simulink model "Pendulo_Invertido"  (R2025b)
settings: Solver=ode45  StartTime=0.0  StopTime=10.0  MaxStep=1e-3  RelTol=1e-3
values from neighbouring files (symbols this model uses):
  alpha = m_p + m_c    (= 2.1)    [Coefficients.m]
  b = 2*zeta_c*omega_p*alpha    [Coefficients.m]
  beta = 2*zeta_p*omega_p*(lambda-mu^2/alpha)    [Coefficients.m]
  F_equilibrium = 1.5*alpha*g*tand(80)    [Coefficients.m]
  g = 9.80665    [Coefficients.m]
  h_c = 0.05    [Coefficients.m]
  l = 0.5    [Coefficients.m]
  lambda = 4/3 * m_p * l^2    (= 0.0333333333333)    [Coefficients.m]
  mu = m_p * l    (= 0.05)    [Coefficients.m]
  x_ref = 0    [Coefficients.m]
libraries: sim3dlib x4, fuzblock x2
settings Model: SimulationMode=accelerator  Creator=barrios14101  LastModifiedBy=admin

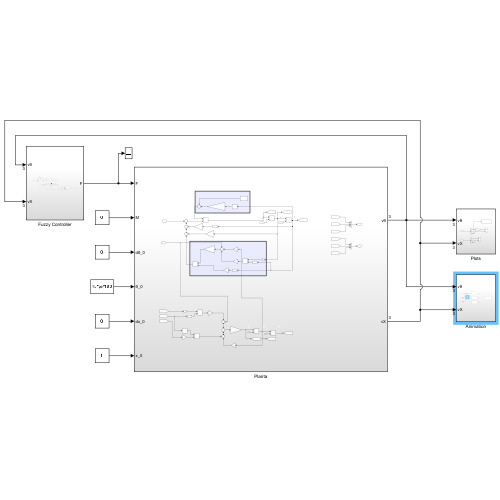
[thumbnail: Simulink's stored preview of the top-level diagram]
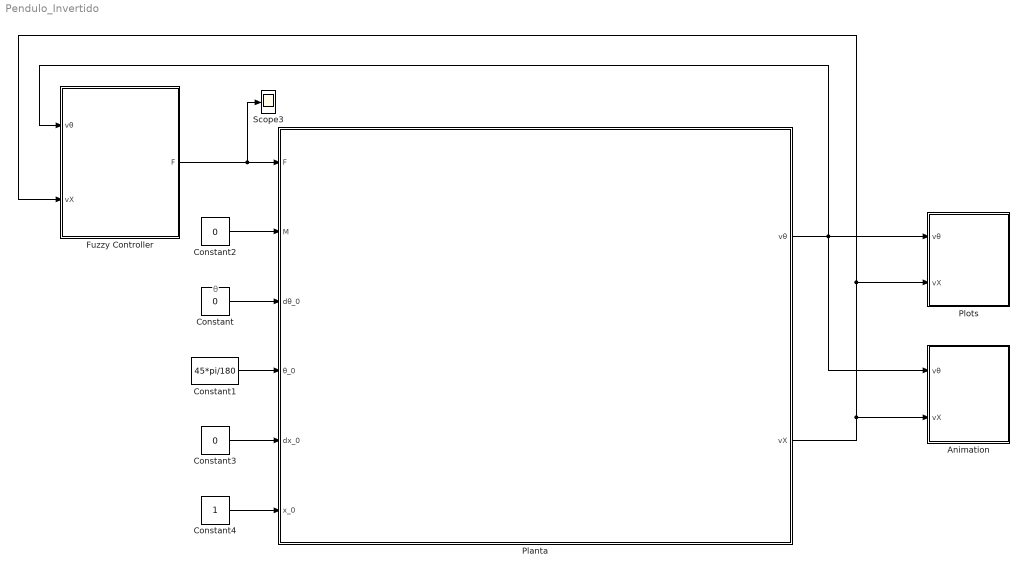
== system Pendulo_Invertido ==
  note: θ
  Animation : Subsystem
  Constant : Constant  Value=0
  Constant1 : Constant  Value=45*pi/180
  Constant2 : Constant  Value=0
  Constant3 : Constant  Value=0
  Constant4 : Constant
  Fuzzy Controller : Subsystem
  Planta : Subsystem
  Plots : Subsystem
  Scope3 : Scope
      settings: ActiveDisplayYMinimum=-600.8821467974509  ActiveDisplayYMaximum=220.63357171688955  DataLoggingDecimation=50  DataLoggingVariableName=ScopeData2
  wires:
  Planta/1(vθ) -> Animation/1(vθ), Plots/1(vθ), Fuzzy Controller/1(vθ)
  Constant/1 -> Planta/3(dθ_0)
  Constant1/1 -> Planta/4(θ_0)
  Planta/2(vX) -> Fuzzy Controller/2(vX), Plots/2(vX), Animation/2(vX)
  Fuzzy Controller/1(F) -> Scope3/1, Planta/1(F)
  Constant2/1 -> Planta/2(M)
  Constant3/1 -> Planta/5(dx_0)
  Constant4/1 -> Planta/6(x_0)

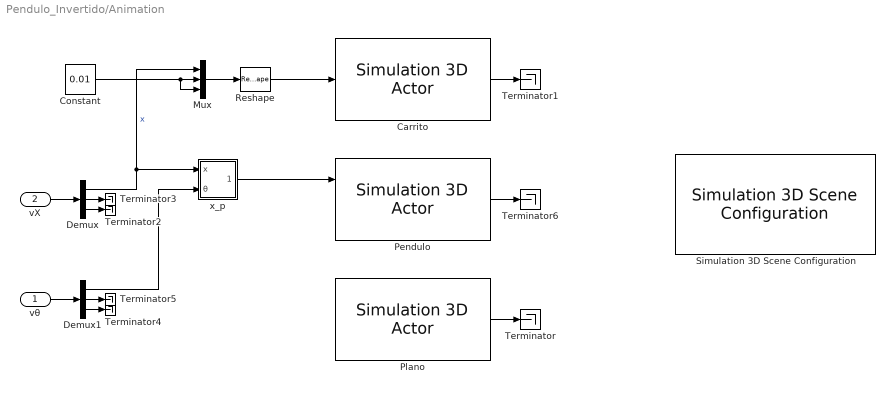
== system Pendulo_Invertido/Animation ==
  vθ : Inport
  vX : Inport  Port=2
  Carrito : sim3dlib/Simulation 3D Actor  Priority=1  ActorName=Carrito  ParentName=Scene Origin  Operation=Create at setup  InitScriptText=|  SampleTime=-1  Translation=[0 0 0]  Rotation=[0 0 0]  Scale=[1 1 1]  InputsText=Carrito.Translation  aMode=5  ActorTag=Carrito  ActorType=Sim3dActor  ID=C
      | createShape(Actor, 'box', [0.5 0.2 0.2]);
      | Actor.Color = [1 0 0];
      | Actor.Physics = false;
      | Actor.Gravity = false;
      | 
      | % Reserved keywords:
      | % - Actor : handle to this actor object
      | % - World : handle to the world object
      | 
      | % Examples:
      | 
      | % Create a primitive geometry (optional)
      | % createShape(Actor, 'box', [1 1 1]);
      | 
      | % Initialize values (optional)
      | % Actor.Physics = true;
      | % Actor.Color = [1 0 0];
  Constant : Constant  Value=0.01
  Demux : Demux  Outputs=3
  Demux1 : Demux  Outputs=3
  Mux : Mux  Inputs=3
  Pendulo : sim3dlib/Simulation 3D Actor  Priority=1  ActorName=Pendulo  ParentName=Scene Origin  Operation=Create at setup  InitScriptText=|  SampleTime=-1  Translation=[0 0 0]  Rotation=[0 0 0]  Scale=[1 1 1]  InputsText=Pendulo.Translation Pendulo.Rotation  aMode=5  ActorTag=Pendulo  ActorType=Sim3dActor  ID=C
      | createShape(Actor, 'cylinder', [0.025 0.025 0.1]);Actor.Color = [1 0 0];
      | Actor.Physics = false;
      | Actor.Gravity = false;
      | 
      | % Reserved keywords:
      | % - Actor : handle to this actor object
      | % - World : handle to the world object
      | 
      | % Examples:
      | 
      | % Create a primitive geometry (optional)
      | % createShape(Actor, 'box', [1 1 1]);
      | 
      | % Initialize values (optional)
      | % Actor.Physics = true;
      | % Actor.Color = [1 0 0];
  Plano : sim3dlib/Simulation 3D Actor  Priority=1  ActorName=Sim3dActor1  ParentName=Scene Origin  Operation=Create at setup  InitScriptText=|  SampleTime=-1  Translation=[0 0 0]  Rotation=[0 0 0]  Scale=[1 1 1]  aMode=5  ActorTag=Sim3dActor1  ActorType=Sim3dActor  ID=1
      | createShape(Actor, 'plane', [5 5 0.1]);
      | Actor.PreciseContacts = true;
  Reshape : Reshape  OutputDimensionality=Column vector (2-D)
  Simulation 3D Scene Configuration : sim3dlib/Simulation 3D Scene Configuration  Priority=0  ProjectFormat=Default Scenes  SceneDesc=Empty scene  ProjectName=C:\Program Files\MATLAB\R2025b\toolbox\shared\sim3d_projects\automotive_project_windows\UE\WindowsNoEditor\VehicleSimulation.exe  ScenePath=/Game/Maps/HwStrght  EnableOpenDRIVE=off  vehTagList={'Carrito';'Custom';'Scene Origin';'Sim3dActor1'}  vehTag=Carrito  AttachedCameraRelativeTranslation=[0 0 0]  FreeCameraDefaultInitialTranslation=[-6, 0, 2]  AttachedCameraRelativeRotation=[0 0 0]  FreeCameraDefaultInitialRotation=[0, -15, 0]  ViewpointName=Custom  FreeCameraInitialTranslation=[0, 0, 0]  ViewpointTranslation=[0 0 0]  FreeCameraInitialRotation=[0, 0, 0]  ViewpointRotation=[0 0 0]  OpVisEn=off  Ts=.02  EnableWindow=on  EnableRemoteAccess=off  EnableWeather=off  SunAzimuth=90  SunAltitude=40.0  EnableGeospatialSun=off  Latitude=0  Longitude=0  Date=2023-01-01  Time=10:30:00  GeoTimeZone=-5.0  SunDaylightSaving=off  wind=1  clouds=10  EnableVolumetricClouds=off  CloudCoverage=0  CloudAltitude=6  fog=0  rain=0  RaindropsEffect=off  SnowDensity=0  EnableGeospatial=off  TilesetSource=Earth terrain  UseTrueOrigin=off  OriginHeight=200  OriginLatitude=40.744652  OriginLongitude=-73.988864  MapStyle=Aerial  AdditionalAssetIDs=[]  UseAdvancedSunSky=off  SolarTime=11  TimeZone=-5  Day=21  Month=9  Year=2022  UseDaylightSavingTime=on  DSTStartDay=10  DSTStartMonth=3  DSTEndDay=3  DSTEndMonth=11  DSTSwitchHour=2  sensorTag=MainCamera1  sensorId=1  sensorName=MainCamera1  mountLoc=Origin  offsetFlag=off  tmountOffset=[0, 0, 0]  rmountOffset=[0, 0, 0]  HorizontalResolution=1280  VerticalResolution=720  HorizontalFOV=60  mountPoint=[0 0 0]  mountOrientation=[0 0 0]  aMode=5  ID=1  GeoTrigger=Inactive  ViewNameList={'Custom'}  ViewTranslationList={'[0 0 0]'}  ViewRotationList={'[0 0 0]'}
      settings: LibrarySourceBlock=sl3dlib/Simulation 3D/Environment/Simulation 3D Scene Configuration
  Terminator{,1..6} (7 alike) : Terminator
  x_p : Subsystem  TreatAsAtomicUnit=on
  wires:
  Plano/1 -> Terminator/1
  Carrito/1 -> Terminator1/1
  vX/1 -> Demux/1
  Demux/3 -> Terminator2/1
  Demux/2 -> Terminator3/1
  Demux1/3 -> Terminator4/1
  Demux1/2 -> Terminator5/1
  vθ/1 -> Demux1/1
  Constant/1 -> Mux/3, Mux/2
  Demux/1 -> Mux/1, x_p/1(x)  "x"
  Mux/1 -> Reshape/1
  Pendulo/1 -> Terminator6/1
  Demux1/1 -> x_p/2(θ)
  x_p/1(vX_p) -> Pendulo/1
  Reshape/1 -> Carrito/1

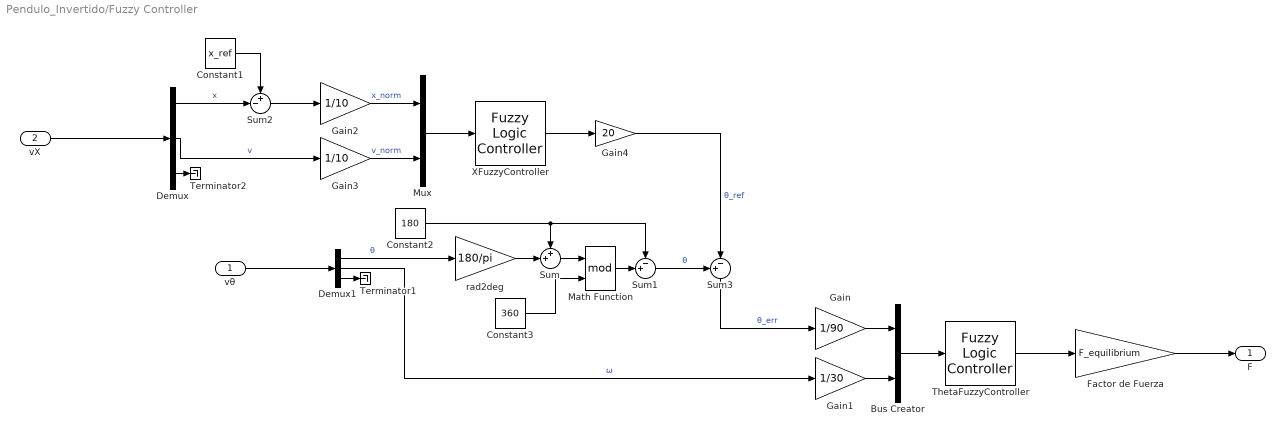
== system Pendulo_Invertido/Fuzzy Controller ==
  vθ : Inport
  vX : Inport  Port=2
  Bus Creator : BusCreator  Inputs=2
  Constant1 : Constant  Value=x_ref
  Constant2 : Constant  Value=180
  Constant3 : Constant  Value=360
  Demux : Demux  Outputs=3
  Demux1 : Demux  Outputs=3
  Factor de Fuerza : Gain  Gain=F_equilibrium
  Gain : Gain  Gain=1/90
  Gain1 : Gain  Gain=1/30
  Gain2 : Gain  Gain=1/10
  Gain3 : Gain  Gain=1/10
  Gain4 : Gain  Gain=20
  Math Function : Math  Operator=mod  OutputSignalType=real
  Mux : Mux  Inputs=2
  Sum : Sum  Inputs=++|
  Sum1 : Sum  Inputs=-+|
  Sum2 : Sum  Inputs=+-|
  Sum3 : Sum  Inputs=+-|
  Terminator1 : Terminator
  Terminator2 : Terminator
  ThetaFuzzyController : fuzblock/Fuzzy Logic  Controller  FIS='ThetaFuzzyController.fis'  OutputSampleNumber=101  DataType=double  UseLookupTable=off  NumBreakpoints=10  FuzzifiedInputs=off  RuleFiringStrengths=off  RuleOutputs=off  AggregatedOutputs=off  SimulateUsing=Interpreted execution  OutOfRangeInputValueMessage=warning  NoRuleFiredMessage=warning  EmptyOutputFuzzySetMessage=warning
  XFuzzyController : fuzblock/Fuzzy Logic  Controller  FIS='XFuzzyController.fis'  OutputSampleNumber=101  DataType=double  UseLookupTable=off  NumBreakpoints=10  FuzzifiedInputs=off  RuleFiringStrengths=off  RuleOutputs=off  AggregatedOutputs=off  SimulateUsing=Interpreted execution  OutOfRangeInputValueMessage=warning  NoRuleFiredMessage=warning  EmptyOutputFuzzySetMessage=warning
  rad2deg : Gain  Gain=180/pi
  F : Outport
  wires:
  ThetaFuzzyController/1 -> Factor de Fuerza/1
  Constant2/1 -> Sum1/1, Sum/1
  rad2deg/1 -> Sum/2
  Math Function/1 -> Sum1/2
  Demux1/2 -> Gain1/1  "ω"
  vθ/1 -> Demux1/1
  Bus Creator/1 -> ThetaFuzzyController/1
  Demux1/1 -> rad2deg/1  "θ"
  Sum/1 -> Math Function/1
  Gain1/1 -> Bus Creator/2
  Constant3/1 -> Math Function/2
  Gain/1 -> Bus Creator/1
  vX/1 -> Demux/1
  Gain2/1 -> Mux/1  "x_norm"
  Demux/2 -> Gain3/1  "v"
  Gain3/1 -> Mux/2  "v_norm"
  Mux/1 -> XFuzzyController/1
  XFuzzyController/1 -> Gain4/1
  Sum1/1 -> Sum3/1  "θ"
  Demux/1 -> Sum2/2  "x"
  Constant1/1 -> Sum2/1
  Sum2/1 -> Gain2/1
  Gain4/1 -> Sum3/2  "θ_ref"
  Sum3/1 -> Gain/1  "θ_err"
  Factor de Fuerza/1 -> F/1
  Demux1/3 -> Terminator1/1
  Demux/3 -> Terminator2/1

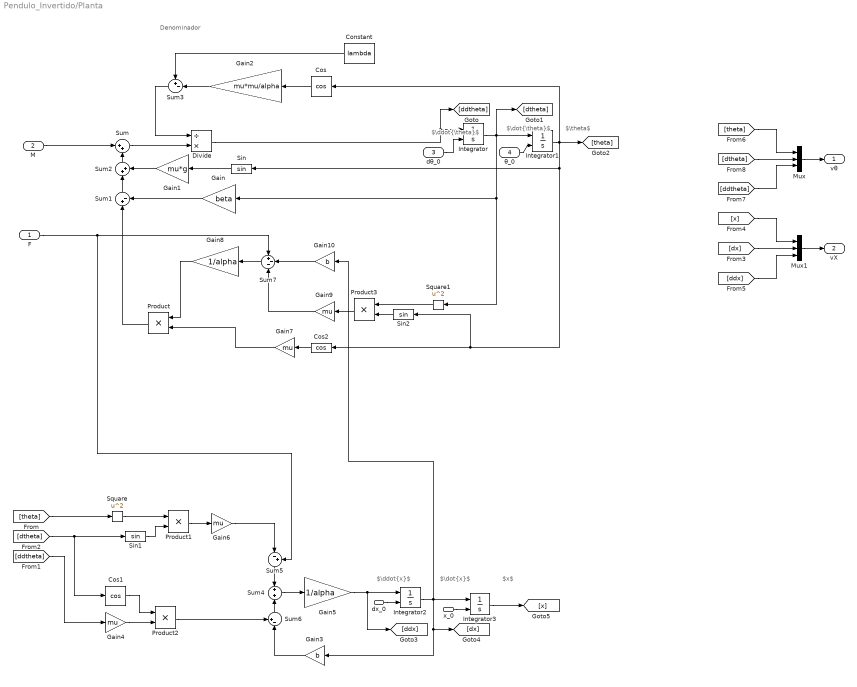
== system Pendulo_Invertido/Planta ==
  note: Denominador
  note: $\ddot{\theta}$
  note: $\dot{\theta}$
  note: $\theta$
  note: $x$
  note: $\ddot{x}$
  note: $\dot{x}$
  F : Inport
  M : Inport  Port=2
  dθ_0 : Inport  Port=3
  θ_0 : Inport  Port=4
  dx_0 : Inport  Port=5
  x_0 : Inport  Port=6
  Constant : Constant  Value=lambda
  Cos : Trigonometry  Operator=cos
  Cos1 : Trigonometry  Operator=cos
  Cos2 : Trigonometry  Operator=cos
  Divide : Product  Inputs=/*
  Gain : Gain  Gain=beta
  Gain1 : Gain  Gain=mu*g
  Gain10 : Gain  Gain=b
  Gain2 : Gain  Gain=mu*mu/alpha
  Gain3 : Gain  Gain=b
  Gain{4,6..7,9} (4 alike) : Gain  Gain=mu
  Gain5 : Gain  Gain=1/alpha
  Gain8 : Gain  Gain=1/alpha
  Integrator : Integrator  InitialConditionSource=external
  Integrator1 : Integrator  InitialConditionSource=external  InitialCondition=pi/12
  Integrator2 : Integrator  InitialConditionSource=external
  Integrator3 : Integrator  InitialConditionSource=external
  Mux : Mux  Inputs=3
  Mux1 : Mux  Inputs=3
  Product{,1..3} (4 alike) : Product
  Sin : Trigonometry
  Sin1 : Trigonometry
  Sin2 : Trigonometry
  Square : Math  Operator=square
  Square1 : Math  Operator=square
  Sum : Sum  Inputs=|++
  Sum1 : Sum  Inputs=|+-
  Sum2 : Sum  Inputs=|++
  Sum3 : Sum  Inputs=+-|
  Sum4 : Sum
  Sum5 : Sum  Inputs=|-+
  Sum6 : Sum  Inputs=+-|
  Sum7 : Sum  Inputs=+--
  vθ : Outport
  vX : Outport  Port=2
  wires:
  Gain8/1 -> Product/1
  Product2/1 -> Sum6/1
  Sum5/1 -> Sum4/1
  Sum6/1 -> Sum4/2
  Constant/1 -> Sum3/1
  Sum1/1 -> Sum2/1
  M/1 -> Sum/1
  Gain3/1 -> Sum6/2
  Gain7/1 -> Product/2
  Sum2/1 -> Sum/2
  F/1 -> Sum5/2, Sum7/1
  Integrator2/1 -> Gain10/1, Integrator3/1, Gain3/1, [dx]
  Gain/1 -> Sum1/2
  [theta] -> Square/1
  Sum7/1 -> Gain8/1
  Square1/1 -> Product3/1
  Gain6/1 -> Sum5/1
  Integrator1/1 -> Sin/1, Sin2/1, Cos2/1, [theta], Cos/1
  Gain4/1 -> Product2/2
  Divide/1 -> [ddtheta], Integrator/1
  Cos/1 -> Gain2/1
  [ddtheta] -> Gain4/1
  Sum/1 -> Divide/2
  Integrator/1 -> [dtheta], Square1/1, Gain/1, Integrator1/1
  Gain1/1 -> Sum2/2
  Gain5/1 -> [ddx], Integrator2/1
  Gain2/1 -> Sum3/2
  Gain9/1 -> Sum7/3
  Cos2/1 -> Gain7/1
  Cos1/1 -> Product2/1
  Sum4/1 -> Gain5/1
  Integrator3/1 -> [x]
  Sin1/1 -> Product1/2
  [dtheta] -> Cos1/1, Sin1/1
  Product3/1 -> Gain9/1
  Gain10/1 -> Sum7/2
  Sum3/1 -> Divide/1
  Product1/1 -> Gain6/1
  Product/1 -> Sum1/1
  Sin2/1 -> Product3/2
  Square/1 -> Product1/1
  Sin/1 -> Gain1/1
  [dtheta] -> Mux/2
  [ddtheta] -> Mux/3
  [x] -> Mux1/1
  [dx] -> Mux1/2
  [ddx] -> Mux1/3
  Mux/1 -> vθ/1
  Mux1/1 -> vX/1
  [theta] -> Mux/1
  dθ_0/1 -> Integrator/2
  θ_0/1 -> Integrator1/2
  dx_0/1 -> Integrator2/2
  x_0/1 -> Integrator3/2

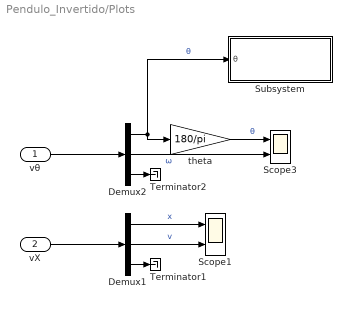
== system Pendulo_Invertido/Plots ==
  vθ : Inport
  vX : Inport  Port=2
  Demux1 : Demux  Outputs=3
  Demux2 : Demux  Outputs=3
  Scope1 : Scope  NumInputPorts=2
      settings: ActiveDisplayYMinimum=-2.2429215830298332  ActiveDisplayYMaximum=1.3603246203366481  DataLoggingDecimation=50
  Scope3 : Scope  NumInputPorts=2
      settings: ActiveDisplayYMinimum=-13.205630471505026  ActiveDisplayYMaximum=51.467292274611673  DataLoggingDecimation=50  DataLoggingVariableName=ScopeData3
  Subsystem : Subsystem
  Terminator1 : Terminator
  Terminator2 : Terminator
  theta : Gain  Gain=180/pi
  wires:
  vθ/1 -> Demux2/1
  Demux1/2 -> Scope1/2  "v"
  Demux1/1 -> Scope1/1  "x"
  vX/1 -> Demux1/1
  Demux2/1 -> theta/1, Subsystem/1(θ)  "θ"
  theta/1 -> Scope3/1  "θ"
  Demux2/2 -> Scope3/2  "ω"
  Demux1/3 -> Terminator1/1
  Demux2/3 -> Terminator2/1

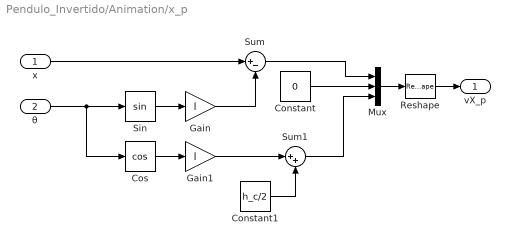
== system Pendulo_Invertido/Animation/x_p ==
  x : Inport
  θ : Inport  Port=2
  Constant : Constant  Value=0
  Constant1 : Constant  Value=h_c/2
  Cos : Trigonometry  Operator=cos
  Gain : Gain  Gain=l
  Gain1 : Gain  Gain=l
  Mux : Mux  Inputs=3
  Reshape : Reshape  OutputDimensionality=Column vector (2-D)
  Sin : Trigonometry
  Sum : Sum  Inputs=|+-
  Sum1 : Sum  Inputs=|++
  vX_p : Outport
  wires:
  θ/1 -> Cos/1, Sin/1
  Sin/1 -> Gain/1
  Gain/1 -> Sum/2
  x/1 -> Sum/1
  Cos/1 -> Gain1/1
  Sum/1 -> Mux/1
  Constant/1 -> Mux/2
  Gain1/1 -> Sum1/1
  Sum1/1 -> Mux/3
  Constant1/1 -> Sum1/2
  Mux/1 -> Reshape/1
  Reshape/1 -> vX_p/1

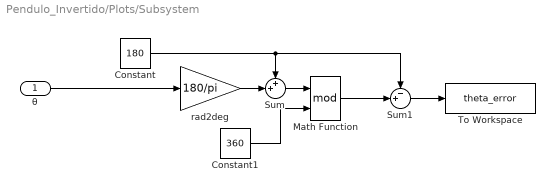
== system Pendulo_Invertido/Plots/Subsystem ==
  θ : Inport
  Constant : Constant  Value=180
  Constant1 : Constant  Value=360
  Math Function : Math  Operator=mod  OutputSignalType=real
  Sum : Sum  Inputs=++|
  Sum1 : Sum  Inputs=-+|
  To Workspace : ToWorkspace  VariableName=theta_error  SaveFormat=Timeseries  SampleTime=-1
  rad2deg : Gain  Gain=180/pi
  wires:
  Math Function/1 -> Sum1/2
  rad2deg/1 -> Sum/2
  Sum/1 -> Math Function/1
  Constant/1 -> Sum1/1, Sum/1
  θ/1 -> rad2deg/1
  Constant1/1 -> Math Function/2
  Sum1/1 -> To Workspace/1
